simulink model "Battery_model"  (R2020a)
settings: Solver=VariableStepAuto  StartTime=0.0  StopTime=3600  RelTol=1e-3
values from neighbouring files (symbols this model uses):
  Cn = 2.3*3600    (= 8280)    [Scribt.m]
  i = 2.3    [Scribt.m]
  OCV = Data(:,2)    [Scribt.m]
  R_Charage = Data(:,3)    [Scribt.m]
  R_DisCharage = Data(:,4)    [Scribt.m]
  SOC = Data(:,1)    [Scribt.m]
settings Model: Creator=eslam  LastModifiedBy=eslam

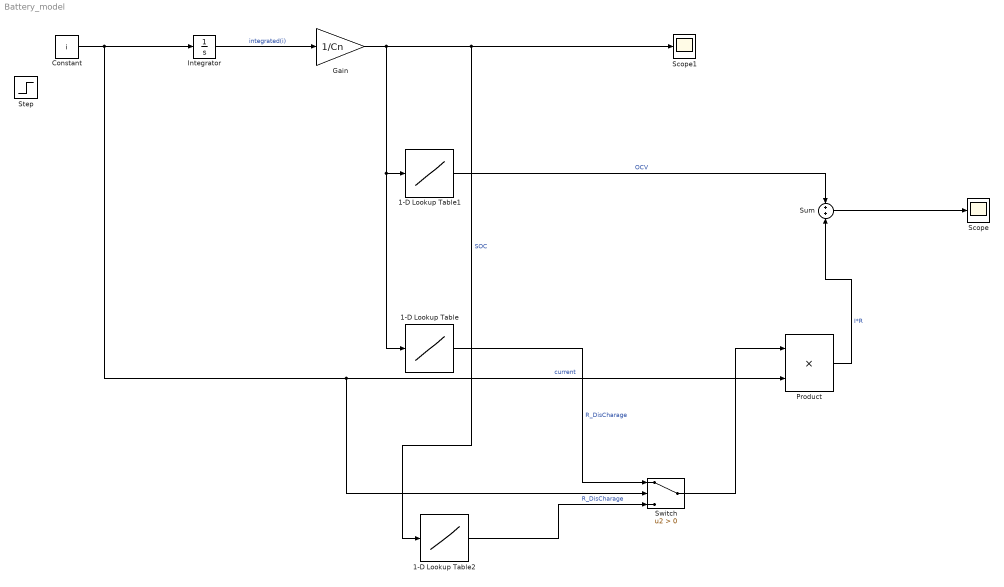
== system Battery_model ==
  1-D Lookup Table : Lookup_n-D  NumberOfTableDimensions=1  BreakpointsForDimension1=SOC  Table=R_DisCharage  InternalRulePriority=Speed  RndMeth=Simplest  InputSameDT=on
  1-D Lookup Table1 : Lookup_n-D  NumberOfTableDimensions=1  BreakpointsForDimension1=SOC  Table=OCV  InternalRulePriority=Speed  RndMeth=Simplest  InputSameDT=on
  1-D Lookup Table2 : Lookup_n-D  NumberOfTableDimensions=1  BreakpointsForDimension1=SOC  Table=R_Charage  InternalRulePriority=Speed  RndMeth=Simplest  InputSameDT=on
  Constant : Constant  Value=i
  Gain : Gain  Gain=1/Cn
  Integrator : Integrator
  Product : Product
  Scope : Scope
  Scope1 : Scope
  Step : Step  SampleTime=0
  Sum : Sum
  Switch : Switch  Criteria=u2 > Threshold
  wires:
  Constant/1 -> Switch/2, Product/2, Integrator/1  "current"
  Integrator/1 -> Gain/1  "integrated(i)"
  Gain/1 -> Scope1/1, 1-D Lookup Table2/1, 1-D Lookup Table/1, 1-D Lookup Table1/1  "SOC"
  1-D Lookup Table/1 -> Switch/1  "R_DisCharage"
  1-D Lookup Table1/1 -> Sum/1  "OCV"
  Product/1 -> Sum/2  "I*R"
  Sum/1 -> Scope/1
  1-D Lookup Table2/1 -> Switch/3  "R_DisCharage"
  Switch/1 -> Product/1
